simulink model "simple_pendulum_simulation"  (R2018a)
settings: Solver=ode45  StartTime=0.0  StopTime=10.0  RelTol=1e-3
settings Model: Creator=Jarvis  LastModifiedBy=Jarvis

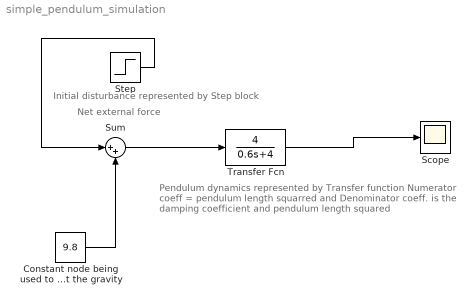
== system simple_pendulum_simulation ==
  note: Net external force
  note: Initial disturbance represented by Step block
  note: Pendulum dynamics represented by Transfer function
      |
      | Numerator coeff = pendulum length squarred and Denominator
      | coeff. is the damping coefficient and pendulum length squared
  Constant node being used to represent the gravity : Constant  Value=9.8
  Scope : Scope
  Step : Step  SampleTime=0
  Sum : Sum  Inputs=|++
  Transfer Fcn : TransferFcn  Numerator=4  Denominator=[0.6 4]
  wires:
  Step/1 -> Sum/1
  Constant node being used to represent the gravity/1 -> Sum/2
  Sum/1 -> Transfer Fcn/1
  Transfer Fcn/1 -> Scope/1
